simulink model "WDS"  (R2022b)
settings: Solver=FixedStepDiscrete  StartTime=0.0  StopTime=T_final  FixedStep=T_sample  RelTol=1e-3
values from neighbouring files (symbols this model uses):
  A_bar_d = readmatrix('A_bar_d.csv')    [Run_model_WDS.m]
  B_bar_d = readmatrix('B_bar_d.csv')    [Run_model_WDS.m]
  C_obsv_d = readmatrix('C_obsv_d.csv')    [Run_model_WDS.m]
  Cm = ones(1,n_states)    [Run_model_WDS.m]
  D_obsv_d = readmatrix('D_obsv_d.csv')    [Run_model_WDS.m]
  H0_perp_full = eye(size(H0_full,1)) - H0_full*H0_full_pinv    [Run_model_WDS.m]
  K = place(A_bar_d,B_bar_d,Pc)    [Run_model_WDS.m]
  Lu = F-A_bar_d.'*H0_full_pinv*H1_full    [Run_model_WDS.m]
  Ly = A_bar_d.'*H0_full_pinv    [Run_model_WDS.m]
  offset = -inv(B_bar_d)*(A_bar_d-eye(n_states))*xd    [Run_model_WDS.m]
  T_sample = 0.01    [Run_model_WDS.m]
  U0 = zeros(n_int,T+1)    [Run_model_WDS.m]
  x0 = zeros(n_states,1)    [Run_model_WDS.m]
  xd = linspace(20,50,n_states)'    [Run_model_WDS.m]
  Y0 = zeros(n_meas,T)    [Run_model_WDS.m]
undefined symbols (not defined in the file or in its folder): H1_full, T_start_opt
libraries: simulink x2
settings Model: Creator=Abelb  LastModifiedBy=Abelb
settings ModelReferenceCC: EnableRefExpFcnMdlSchedulingChecks=on

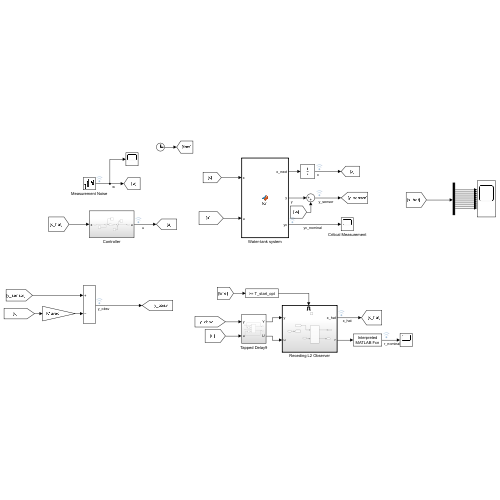
[thumbnail: Simulink's stored preview of the top-level diagram]
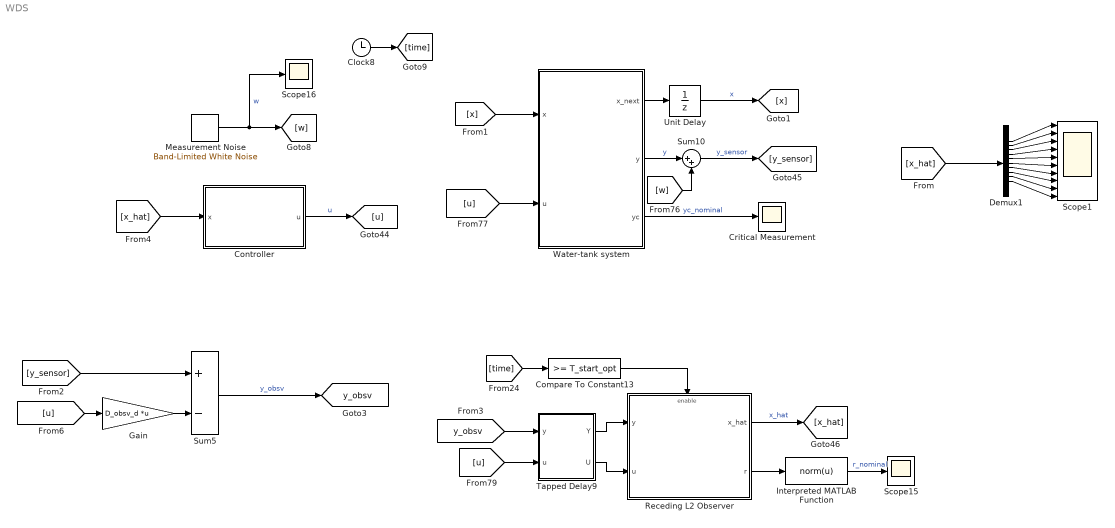
== system WDS ==
  Clock8 : Clock
  Compare To Constant13 : simulink/Logic and Bit Operations/Compare To Constant  relop=>=  const=T_start_opt  OutDataTypeStr=boolean
  Controller : Subsystem
  Critical Measurement : Scope
  Demux1 : Demux  Outputs=n_states
  Gain : Gain  Gain=D_obsv_d  Multiplication=Matrix(K*u) (u vector)
  Interpreted MATLAB Function : MATLABFcn  MATLABFcn=norm(u)
  Measurement Noise : simulink/Sources/Band-Limited White Noise  Cov=[1e-7]  Ts=T_sample  seed=[23341]
  Receding L2 Observer : Subsystem
  Scope1 : Scope  NumInputPorts=10
  Scope15 : Scope
  Scope16 : Scope
  Sum10 : Sum  Inputs=|++
  Sum5 : Sum  Inputs=+-
  Tapped Delay9 : Subsystem
  Unit Delay : UnitDelay  InitialCondition=x0  SampleTime=-1  HasFrameUpgradeWarning=on
  Water-tank system : MATLAB Function  TreatAsAtomicUnit=on
  tag scope: y_obsv=global
  wires:
  [y_obsv] -> Tapped Delay9/1(y)
  Measurement Noise/1 -> Scope16/1, [w]  "w"
  Receding L2 Observer/2(r) -> Interpreted MATLAB Function/1
  Unit Delay/1 -> [x]  "x"
  Water-tank system/3(yc) -> Critical Measurement/1  "yc_nominal"
  Interpreted MATLAB Function/1 -> Scope15/1  "r_nominal"
  [w] -> Sum10/2
  [x_hat] -> Controller/1(x)
  Compare To Constant13/1 -> Receding L2 Observer/Enable
  [time] -> Compare To Constant13/1
  Receding L2 Observer/1(x_hat) -> [x_hat]  "x_hat"
  [u] -> Water-tank system/2(u)
  Sum10/1 -> [y_sensor]  "y_sensor"
  Tapped Delay9/1(Y) -> Receding L2 Observer/1(y)
  Controller/1(u) -> [u]  "u"
  Tapped Delay9/2(U) -> Receding L2 Observer/2(u)
  Water-tank system/2(y) -> Sum10/1  "y"
  [u] -> Tapped Delay9/2(u)
  Water-tank system/1(x_next) -> Unit Delay/1
  [y_sensor] -> Sum5/1
  [u] -> Gain/1
  Gain/1 -> Sum5/2
  Sum5/1 -> [y_obsv]  "y_obsv"
  Demux1/1 -> Scope1/1
  Demux1/3 -> Scope1/3
  Demux1/9 -> Scope1/9
  Demux1/6 -> Scope1/6
  Demux1/5 -> Scope1/5
  Demux1/4 -> Scope1/4
  Demux1/8 -> Scope1/8
  Demux1/2 -> Scope1/2
  Demux1/7 -> Scope1/7
  Demux1/10 -> Scope1/10
  [x_hat] -> Demux1/1
  Clock8/1 -> [time]
  [x] -> Water-tank system/1(x)

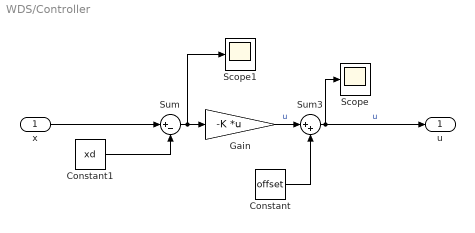
== system WDS/Controller ==
  x : Inport
  Constant : Constant  Value=offset
  Constant1 : Constant  Value=xd
  Gain : Gain  Gain=-K  Multiplication=Matrix(K*u) (u vector)
  Scope : Scope
  Scope1 : Scope
  Sum : Sum  Inputs=|+-
  Sum3 : Sum  Inputs=|++
  u : Outport
  wires:
  Sum3/1 -> u/1, Scope/1  "u"
  Constant/1 -> Sum3/2
  Constant1/1 -> Sum/2
  Gain/1 -> Sum3/1  "u"
  Sum/1 -> Scope1/1, Gain/1
  x/1 -> Sum/1

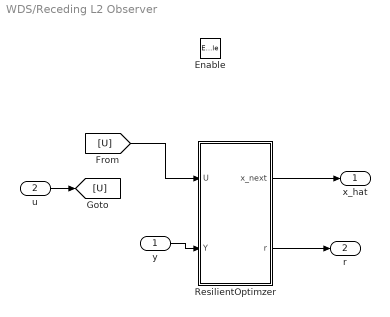
== system WDS/Receding L2 Observer ==
  y : Inport
  u : Inport  Port=2
  Enable : EnablePort
  ResilientOptimzer : MATLAB Function  TreatAsAtomicUnit=on
  x_hat : Outport
  r : Outport  Port=2
  wires:
  u/1 -> [U]
  y/1 -> ResilientOptimzer/2(Y)
  [U] -> ResilientOptimzer/1(U)
  ResilientOptimzer/1(x_next) -> x_hat/1
  ResilientOptimzer/2(r) -> r/1

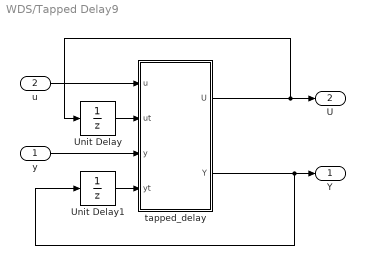
== system WDS/Tapped Delay9 ==
  y : Inport
  u : Inport  Port=2
  Unit Delay : UnitDelay  InitialCondition=U0  SampleTime=-1  HasFrameUpgradeWarning=on
  Unit Delay1 : UnitDelay  InitialCondition=Y0  SampleTime=-1  HasFrameUpgradeWarning=on
  tapped_delay : MATLAB Function  TreatAsAtomicUnit=on
  Y : Outport
  U : Outport  Port=2
  wires:
  u/1 -> tapped_delay/1(u)
  y/1 -> tapped_delay/3(y)
  tapped_delay/1(U) -> Unit Delay/1, U/1
  tapped_delay/2(Y) -> Unit Delay1/1, Y/1
  Unit Delay/1 -> tapped_delay/2(ut)
  Unit Delay1/1 -> tapped_delay/4(yt)

== matlab function WDS/Receding L2 Observer/ResilientOptimzer ==
  data: x_next output; U input; Y input; Ly parameter; Lu parameter; H0_perp_full parameter; H1_full parameter; r output
function [x_next,r]  = fcn(U,Y, Ly, Lu,H0_perp_full, H1_full)


u_local = U(:,1:end-1);
% vectorized
u = u_local(:);
y = Y(:);

x_next = zeros(10,1);
x_next(:) = Ly*y + Lu*u;

r = H0_perp_full*(y-H1_full*u);

== matlab function WDS/Tapped Delay9/tapped_delay ==
  data: u input; U output; ut input; y input; yt input; Y output
function [U,Y] = fcn(u,ut,y,yt)
%% tapped_delay_array
% shift columns from tapped matrix to the left and appends most recent
% vector to the last column
%%% input
ut(:,1:end-1) = ut(:,2:end);
ut(:,end) = u;
U = ut;
%%% output
yt(:,1:end-1) = yt(:,2:end);
yt(:,end) = y;
Y = yt;

== matlab function WDS/Water-tank system ==
  data: x input; x_next output; u input; y output; A_bar_d parameter; C_obsv_d parameter; B_bar_d parameter; D_obsv_d parameter; yc output; Cm parameter
function [x_next,y,yc] = fcn(x,u,A_bar_d,C_obsv_d,B_bar_d,D_obsv_d,Cm)
% Discrete state-space model for system

x_next = A_bar_d*x + B_bar_d*u ;

y = C_obsv_d*x + D_obsv_d*u;

% critical measurements
yc = Cm*x;
